simulink model "acdcmg_sim8_1_sm_grid_simulation"  (R2019b)
settings: Solver=ode8  StartTime=0.0  StopTime=0.5  FixedStep=4e-05  MaxStep=1e-2  RelTol=1e-3
PreLoadFcn:
  | Set_parameters_R2018
InitFcn:
  | Set_parameters_R2018
undefined symbols (not defined in the file or in its folder): D1, Delta, dis11, dis12, dis2, dis3, dis4, dis5, dis6, DiscIntNeverNeededParam, fn, Fnom, Ion, Lithium, max_min, P_Load_3, Pnom_T1, Pnom_T2, Pnom_T3, Ql_Load_3, R_Load_9, R_Load_DC, Rl, Rls, Ts, Ts_Control, Ts_Power, Ts_PV, V1_LL_T3, Vmin_mppt, VnInv, Vnom_DC, Vnom_Diesel, Vnom_prim, Vnom_sec, Vnom_ter_AC_DC, Xl, Xls
libraries: powerlib x136, powerlib_meascontrol x67, opal_lib x24, artemis x7, simulink x7, powerlib_extras x5, electricdrivelib x1, eeSinusoidalMeasurementV2 x1, re_lib x1
(part 2 of 4)

== system acdcmg_sim8_1_sm_grid_simulation/SM_Grid_Simulation/Bus_1 ==
  Mux : Mux  Inputs=2
  "Power (3ph, Instantaneous)" : powerlib_meascontrol/Measurements/Power (3ph, Instantaneous)
  Power Factor Block1 : Subsystem  mask(Power Factor Block){Freq=Fnom, Vinit=[0, 0], Iinit=[0, 0], Ts=0}
      mask prompts: Freq "Fundamental frequency (Hz):"; Vinit "Voltage initial input [ Mag, Phase (degrees) ]:"; Iinit "Current initial input [ Mag, Phase (degrees) ]:"; Ts "Sample time:"
      mask help:
      | Power Factor Block developed by Dr Rodney Tan
      | Version 1.01 (Aug 2016)
      |
      | Compute power factor and phase angle of AC circuit voltage-current pair at fundamental frequency.
      |
      | The computation is based on Power block and Complex number function block.
      |
      | For the first cycle of simulation, the outputs are held constant to the powers computed for the Voltage initial input and Current initial input parameters.
      mask Help:
      | <b>Fundamental Frequency (Hz)</b>
      | Specify the measurement fundamental frequency, in hertz, of the input signal.
      | 
      | <b>Voltage initial input [ Mag, Phase (degrees) ]</b>
      | Specify the voltage initial magnitude and phase to set a constant output for the first cycle of simulation.
      | 
      | <b>Current initial input [ Mag, Phase (degrees) ]</b>
      | Specify the current initial magnitude and phase to set a constant output for the first cycle of simulation.
      | 
      | <b>Sample Time</b>
      | Specify the sample time of the block, in seconds. Set to 0 to implement a continuous block.
      mask TypeOptions Freq: Power/Freq
      mask TypeOptions Vinit: Power/Vinit
      mask TypeOptions Iinit: Power/Iinit
      mask TypeOptions Ts: Power/Ts
  "Means_Bus1      " : Outport  VectorParamsAs1DForOutWhenUnconnected=off
  tag scope: Bus1_Iabc=global, Bus1_P=global, Bus1_Q=global, Bus1_Vabc=global
  wires:
  [IabcLL_Bus_1] -> "Power (3ph, Instantaneous)"/2, Power Factor Block1/2(Iabc), Mux/2  "Iabc"
  Mux/1 -> "Means_Bus1      "/1
  Power Factor Block1/2("Iabc y Iabc ") -> [Bus1_Iabc]
  Power Factor Block1/1("Vabc y Vabc ") -> [Bus1_Vabc]
  [VabcLL_Bus_1] -> Power Factor Block1/1(Vabc), "Power (3ph, Instantaneous)"/1, Mux/1  "Vabc"
  "Power (3ph, Instantaneous)"/1 -> [Bus1_P]
  "Power (3ph, Instantaneous)"/2 -> [Bus1_Q]

== system acdcmg_sim8_1_sm_grid_simulation/SM_Grid_Simulation/Bus_14 1 ==
  " r1_ L13" : Constant  Value=Rl
  Active powers losses A : Display
      settings: Format=bank
  Active powers losses B : Display
      settings: Format=bank
  Active powers losses c : Display
      settings: Format=bank
  Math Function : Math  Operator=square  SaturateOnIntegerOverflow=on
  Math Function1 : Math  Operator=square  SaturateOnIntegerOverflow=on
  Math Function2 : Math  Operator=square  SaturateOnIntegerOverflow=on
  Mux : Mux  Inputs=3
  Product : Product
  Product1 : Product
  Product2 : Product
  RMS1 : powerlib_meascontrol/Measurements/RMS  TrueRMS=on  Freq=60  RMSInit=0  Ts=0
  RMS2 : powerlib_meascontrol/Measurements/RMS  TrueRMS=on  Freq=60  RMSInit=0  Ts=0
  RMS3 : powerlib_meascontrol/Measurements/RMS  TrueRMS=on  Freq=60  RMSInit=0  Ts=0
  W_to_kW : Gain  Gain=1e-3
  W_to_kW1 : Gain  Gain=1e-3
  W_to_kW2 : Gain  Gain=1e-3
  tag scope: Bus_14_1_LineA_Ploss=global, Bus_14_1_LineB_Ploss=global, Bus_14_1_LineC_Ploss=global, Power_Losse_abc_L1=global
  wires:
  Math Function/1 -> Product/2
  [Ia_L1] -> RMS2/1
  Math Function1/1 -> Product1/2
  [Ib_L1] -> RMS1/1
  Math Function2/1 -> Product2/2
  " r1_ L13"/1 -> Product2/1, Product1/1, Product/1
  [Ic_L1] -> RMS3/1
  Product/1 -> W_to_kW/1
  Product2/1 -> W_to_kW2/1
  Product1/1 -> W_to_kW1/1
  RMS2/1 -> Math Function/1
  RMS1/1 -> Math Function1/1
  RMS3/1 -> Math Function2/1
  W_to_kW/1 -> [Bus_14_1_LineA_Ploss], Mux/1, Active powers losses A/1  "D_Pa_kW"
  W_to_kW1/1 -> [Bus_14_1_LineB_Ploss], Mux/2, Active powers losses B/1  "D_Pb_kW"
  W_to_kW2/1 -> Active powers losses c/1, [Bus_14_1_LineC_Ploss], Mux/3  "D_Pc_kW"
  Mux/1 -> [Power_Losse_abc_L1]

== system acdcmg_sim8_1_sm_grid_simulation/SM_Grid_Simulation/Bus_14 2 ==
  " r1_ L13" : Constant  Value=Rls
  Active powers losses A : Display
      settings: Format=bank
  Active powers losses B : Display
      settings: Format=bank
  Active powers losses c : Display
      settings: Format=bank
  Math Function : Math  Operator=square  SaturateOnIntegerOverflow=on
  Math Function1 : Math  Operator=square  SaturateOnIntegerOverflow=on
  Math Function2 : Math  Operator=square  SaturateOnIntegerOverflow=on
  Mux : Mux  Inputs=3
  Product : Product
  Product1 : Product
  Product2 : Product
  RMS1 : powerlib_meascontrol/Measurements/RMS  TrueRMS=on  Freq=60  RMSInit=0  Ts=0
  RMS2 : powerlib_meascontrol/Measurements/RMS  TrueRMS=on  Freq=60  RMSInit=0  Ts=0
  RMS3 : powerlib_meascontrol/Measurements/RMS  TrueRMS=on  Freq=60  RMSInit=0  Ts=0
  W_to_kW : Gain  Gain=1e-3
  W_to_kW1 : Gain  Gain=1e-3
  W_to_kW2 : Gain  Gain=1e-3
  tag scope: Bus_14_2_LineA_Ploss=global, Bus_14_2_LineB_Ploss=global, Bus_14_2_LineC_Ploss=global, Power_Losse_abc_L2=global
  wires:
  Math Function/1 -> Product/2
  [Ia_L2] -> RMS2/1
  Math Function1/1 -> Product1/2
  [Ib_L2] -> RMS1/1
  Math Function2/1 -> Product2/2
  " r1_ L13"/1 -> Product2/1, Product1/1, Product/1
  [Ic_L2] -> RMS3/1
  Product/1 -> W_to_kW/1
  Product2/1 -> W_to_kW2/1
  Product1/1 -> W_to_kW1/1
  RMS2/1 -> Math Function/1
  RMS1/1 -> Math Function1/1
  RMS3/1 -> Math Function2/1
  W_to_kW/1 -> [Bus_14_2_LineA_Ploss], Mux/1, Active powers losses A/1  "D_Pa_kW"
  W_to_kW1/1 -> [Bus_14_2_LineB_Ploss], Mux/2, Active powers losses B/1  "D_Pb_kW"
  W_to_kW2/1 -> Active powers losses c/1, [Bus_14_2_LineC_Ploss], Mux/3  "D_Pc_kW"
  Mux/1 -> [Power_Losse_abc_L2]

== system acdcmg_sim8_1_sm_grid_simulation/SM_Grid_Simulation/Bus_14 3 ==
  " r1_ L13" : Constant  Value=Rl
  Active powers losses A : Display  Commented=on
      settings: Format=bank
  Active powers losses B : Display  Commented=on
      settings: Format=bank
  Active powers losses c : Display  Commented=on
      settings: Format=bank
  "Delta Pabc " : Scope  NumInputPorts=4
  Math Function : Math  Operator=square  SaturateOnIntegerOverflow=on
  Math Function1 : Math  Operator=square  SaturateOnIntegerOverflow=on
  Math Function2 : Math  Operator=square  SaturateOnIntegerOverflow=on
  Mux : Mux  Inputs=3
  Product : Product
  Product1 : Product
  Product2 : Product
  RMS1 : powerlib_meascontrol/Measurements/RMS  TrueRMS=on  Freq=60  RMSInit=0  Ts=0
  RMS2 : powerlib_meascontrol/Measurements/RMS  TrueRMS=on  Freq=60  RMSInit=0  Ts=0
  RMS3 : powerlib_meascontrol/Measurements/RMS  TrueRMS=on  Freq=60  RMSInit=0  Ts=0
  W_to_kW : Gain  Gain=1e-3
  W_to_kW1 : Gain  Gain=1e-3
  W_to_kW2 : Gain  Gain=1e-3
  tag scope: Bus_14_3_LineA_Ploss=global, Bus_14_3_LineB_Ploss=global, Bus_14_3_LineC_Ploss=global, Power_Losse_abc_L3=global
  wires:
  Math Function/1 -> Product/2
  [Ia_L3] -> RMS2/1
  Math Function1/1 -> Product1/2
  [Ib_L3] -> RMS1/1
  Math Function2/1 -> Product2/2
  " r1_ L13"/1 -> Product2/1, Product1/1, Product/1
  [Ic_L3] -> RMS3/1
  Product/1 -> W_to_kW/1
  Product2/1 -> W_to_kW2/1
  Product1/1 -> W_to_kW1/1
  RMS2/1 -> Math Function/1
  RMS1/1 -> Math Function1/1
  RMS3/1 -> Math Function2/1
  W_to_kW/1 -> Mux/1, [Bus_14_3_LineA_Ploss], Active powers losses A/1  "D_Pa_kW"
  W_to_kW1/1 -> Mux/2, [Bus_14_3_LineB_Ploss], Active powers losses B/1  "D_Pb_kW"
  W_to_kW2/1 -> Active powers losses c/1, Mux/3, [Bus_14_3_LineC_Ploss]  "D_Pc_kW"
  Mux/1 -> [Power_Losse_abc_L3]

== system acdcmg_sim8_1_sm_grid_simulation/SM_Grid_Simulation/Bus_14 4 ==
  " r1_ L13" : Constant  Value=Rls
  Active powers losses A : Display
      settings: Format=bank
  Active powers losses B : Display
      settings: Format=bank
  Active powers losses c : Display
      settings: Format=bank
  Math Function : Math  Operator=square  SaturateOnIntegerOverflow=on
  Math Function1 : Math  Operator=square  SaturateOnIntegerOverflow=on
  Math Function2 : Math  Operator=square  SaturateOnIntegerOverflow=on
  Mux : Mux  Inputs=3
  Product : Product
  Product1 : Product
  Product2 : Product
  RMS1 : powerlib_meascontrol/Measurements/RMS  TrueRMS=on  Freq=60  RMSInit=0  Ts=0
  RMS2 : powerlib_meascontrol/Measurements/RMS  TrueRMS=on  Freq=60  RMSInit=0  Ts=0
  RMS3 : powerlib_meascontrol/Measurements/RMS  TrueRMS=on  Freq=60  RMSInit=0  Ts=0
  W_to_kW : Gain  Gain=1e-3
  W_to_kW1 : Gain  Gain=1e-3
  W_to_kW2 : Gain  Gain=1e-3
  tag scope: Bus_14_4_LineA_Ploss=global, Bus_14_4_LineB_Ploss=global, Bus_14_4_LineC_Ploss=global, Power_Losse_abc_L4=global
  wires:
  Math Function/1 -> Product/2
  [Ia_L4] -> RMS2/1
  Math Function1/1 -> Product1/2
  [Ib_L4] -> RMS1/1
  Math Function2/1 -> Product2/2
  " r1_ L13"/1 -> Product2/1, Product1/1, Product/1
  [Ic_L4] -> RMS3/1
  Product/1 -> W_to_kW/1
  Product2/1 -> W_to_kW2/1
  Product1/1 -> W_to_kW1/1
  RMS2/1 -> Math Function/1
  RMS1/1 -> Math Function1/1
  RMS3/1 -> Math Function2/1
  W_to_kW/1 -> Mux/1, [Bus_14_4_LineA_Ploss], Active powers losses A/1  "D_Pa_kW"
  W_to_kW1/1 -> Mux/2, [Bus_14_4_LineB_Ploss], Active powers losses B/1  "D_Pb_kW"
  W_to_kW2/1 -> Active powers losses c/1, [Bus_14_4_LineC_Ploss], Mux/3  "D_Pc_kW"
  Mux/1 -> [Power_Losse_abc_L4]

== system acdcmg_sim8_1_sm_grid_simulation/SM_Grid_Simulation/Bus_14 5 ==
  " r1_ L13" : Constant  Value=Rls
  Active powers losses A : Display
      settings: Format=bank
  Active powers losses B : Display
      settings: Format=bank
  Active powers losses c : Display
      settings: Format=bank
  Math Function : Math  Operator=square  SaturateOnIntegerOverflow=on
  Math Function1 : Math  Operator=square  SaturateOnIntegerOverflow=on
  Math Function2 : Math  Operator=square  SaturateOnIntegerOverflow=on
  Mux : Mux  Inputs=3
  Product : Product
  Product1 : Product
  Product2 : Product
  RMS1 : powerlib_meascontrol/Measurements/RMS  TrueRMS=on  Freq=60  RMSInit=0  Ts=0
  RMS2 : powerlib_meascontrol/Measurements/RMS  TrueRMS=on  Freq=60  RMSInit=0  Ts=0
  RMS3 : powerlib_meascontrol/Measurements/RMS  TrueRMS=on  Freq=60  RMSInit=0  Ts=0
  W_to_kW : Gain  Gain=1e-3
  W_to_kW1 : Gain  Gain=1e-3
  W_to_kW2 : Gain  Gain=1e-3
  tag scope: Bus_14_5_LineA_Ploss=global, Bus_14_5_LineB_Ploss=global, Bus_14_5_LineC_Ploss=global, Power_Losse_abc_L5=global
  wires:
  Math Function/1 -> Product/2
  [Ia_L5] -> RMS2/1
  Math Function1/1 -> Product1/2
  [Ib_L5] -> RMS1/1
  Math Function2/1 -> Product2/2
  " r1_ L13"/1 -> Product2/1, Product1/1, Product/1
  [Ic_L5] -> RMS3/1
  Product/1 -> W_to_kW/1
  Product2/1 -> W_to_kW2/1
  Product1/1 -> W_to_kW1/1
  RMS2/1 -> Math Function/1
  RMS1/1 -> Math Function1/1
  RMS3/1 -> Math Function2/1
  W_to_kW/1 -> [Bus_14_5_LineA_Ploss], Mux/1, Active powers losses A/1  "D_Pa_kW"
  W_to_kW1/1 -> [Bus_14_5_LineB_Ploss], Mux/2, Active powers losses B/1  "D_Pb_kW"
  W_to_kW2/1 -> Active powers losses c/1, [Bus_14_5_LineC_Ploss], Mux/3  "D_Pc_kW"
  Mux/1 -> [Power_Losse_abc_L5]

== system acdcmg_sim8_1_sm_grid_simulation/SM_Grid_Simulation/Bus_14 6 ==
  " r1_ L13" : Constant  Value=Rls
  Active powers losses A : Display
      settings: Format=bank
  Active powers losses B : Display
      settings: Format=bank
  Active powers losses c : Display
      settings: Format=bank
  Math Function : Math  Operator=square  SaturateOnIntegerOverflow=on
  Math Function1 : Math  Operator=square  SaturateOnIntegerOverflow=on
  Math Function2 : Math  Operator=square  SaturateOnIntegerOverflow=on
  Mux : Mux  Inputs=3
  Product : Product
  Product1 : Product
  Product2 : Product
  RMS1 : powerlib_meascontrol/Measurements/RMS  TrueRMS=on  Freq=60  RMSInit=0  Ts=0
  RMS2 : powerlib_meascontrol/Measurements/RMS  TrueRMS=on  Freq=60  RMSInit=0  Ts=0
  RMS3 : powerlib_meascontrol/Measurements/RMS  TrueRMS=on  Freq=60  RMSInit=0  Ts=0
  W_to_kW : Gain  Gain=1e-3
  W_to_kW1 : Gain  Gain=1e-3
  W_to_kW2 : Gain  Gain=1e-3
  tag scope: Bus_14_6_LineA_Ploss=global, Bus_14_6_LineB_Ploss=global, Bus_14_6_LineC_Ploss=global, Power_Losse_abc_L6=global
  wires:
  Math Function/1 -> Product/2
  [Ia_L6] -> RMS2/1
  Math Function1/1 -> Product1/2
  [Ib_L6] -> RMS1/1
  Math Function2/1 -> Product2/2
  " r1_ L13"/1 -> Product2/1, Product1/1, Product/1
  [Ic_L6] -> RMS3/1
  Product/1 -> W_to_kW/1
  Product2/1 -> W_to_kW2/1
  Product1/1 -> W_to_kW1/1
  RMS2/1 -> Math Function/1
  RMS1/1 -> Math Function1/1
  RMS3/1 -> Math Function2/1
  W_to_kW/1 -> [Bus_14_6_LineA_Ploss], Mux/1, Active powers losses A/1  "D_Pa_kW"
  W_to_kW1/1 -> [Bus_14_6_LineB_Ploss], Mux/2, Active powers losses B/1  "D_Pb_kW"
  W_to_kW2/1 -> Active powers losses c/1, [Bus_14_6_LineC_Ploss], Mux/3  "D_Pc_kW"
  Mux/1 -> [Power_Losse_abc_L6]

== system acdcmg_sim8_1_sm_grid_simulation/SM_Grid_Simulation/Bus_14 7 ==
  " r1_ L13" : Constant  Value=Rls
  Active powers losses A : Display
      settings: Format=bank
  Active powers losses B : Display
      settings: Format=bank
  Active powers losses c : Display
      settings: Format=bank
  Math Function : Math  Operator=square  SaturateOnIntegerOverflow=on
  Math Function1 : Math  Operator=square  SaturateOnIntegerOverflow=on
  Math Function2 : Math  Operator=square  SaturateOnIntegerOverflow=on
  Mux : Mux  Inputs=3
  Product : Product
  Product1 : Product
  Product2 : Product
  RMS1 : powerlib_meascontrol/Measurements/RMS  TrueRMS=on  Freq=60  RMSInit=0  Ts=0
  RMS2 : powerlib_meascontrol/Measurements/RMS  TrueRMS=on  Freq=60  RMSInit=0  Ts=0
  RMS3 : powerlib_meascontrol/Measurements/RMS  TrueRMS=on  Freq=60  RMSInit=0  Ts=0
  W_to_kW : Gain  Gain=1e-3
  W_to_kW1 : Gain  Gain=1e-3
  W_to_kW2 : Gain  Gain=1e-3
  tag scope: Bus_14_7_LineA_Ploss=global, Bus_14_7_LineB_Ploss=global, Bus_14_7_LineC_Ploss=global, Power_Losse_abc_L7=global
  wires:
  Math Function/1 -> Product/2
  [Ia_L7] -> RMS2/1
  Math Function1/1 -> Product1/2
  [Ib_L7] -> RMS1/1
  Math Function2/1 -> Product2/2
  " r1_ L13"/1 -> Product2/1, Product1/1, Product/1
  [Ic_L7] -> RMS3/1
  Product/1 -> W_to_kW/1
  Product2/1 -> W_to_kW2/1
  Product1/1 -> W_to_kW1/1
  RMS2/1 -> Math Function/1
  RMS1/1 -> Math Function1/1
  RMS3/1 -> Math Function2/1
  W_to_kW/1 -> [Bus_14_7_LineA_Ploss], Mux/1, Active powers losses A/1  "D_Pa_kW"
  W_to_kW1/1 -> [Bus_14_7_LineB_Ploss], Mux/2, Active powers losses B/1  "D_Pb_kW"
  W_to_kW2/1 -> Active powers losses c/1, [Bus_14_7_LineC_Ploss], Mux/3  "D_Pc_kW"
  Mux/1 -> [Power_Losse_abc_L7]

== system acdcmg_sim8_1_sm_grid_simulation/SM_Grid_Simulation/Bus_2 ==
  "Power (3ph, Instantaneous)" : powerlib_meascontrol/Measurements/Power (3ph, Instantaneous)
  Power Factor Block1 : Subsystem  mask(Power Factor Block){Freq=Fnom, Vinit=[0, 0], Iinit=[0, 0], Ts=0}
      mask prompts: Freq "Fundamental frequency (Hz):"; Vinit "Voltage initial input [ Mag, Phase (degrees) ]:"; Iinit "Current initial input [ Mag, Phase (degrees) ]:"; Ts "Sample time:"
      mask help:
      | Power Factor Block developed by Dr Rodney Tan
      | Version 1.01 (Aug 2016)
      |
      | Compute power factor and phase angle of AC circuit voltage-current pair at fundamental frequency.
      |
      | The computation is based on Power block and Complex number function block.
      |
      | For the first cycle of simulation, the outputs are held constant to the powers computed for the Voltage initial input and Current initial input parameters.
      mask Help:
      | <b>Fundamental Frequency (Hz)</b>
      | Specify the measurement fundamental frequency, in hertz, of the input signal.
      | 
      | <b>Voltage initial input [ Mag, Phase (degrees) ]</b>
      | Specify the voltage initial magnitude and phase to set a constant output for the first cycle of simulation.
      | 
      | <b>Current initial input [ Mag, Phase (degrees) ]</b>
      | Specify the current initial magnitude and phase to set a constant output for the first cycle of simulation.
      | 
      | <b>Sample Time</b>
      | Specify the sample time of the block, in seconds. Set to 0 to implement a continuous block.
      mask TypeOptions Freq: Power/Freq
      mask TypeOptions Vinit: Power/Vinit
      mask TypeOptions Iinit: Power/Iinit
      mask TypeOptions Ts: Power/Ts
  tag scope: Bus2_Iabc=global, Bus2_P=global, Bus2_Q=global, Bus2_Vabc=global
  wires:
  [IabcLL_Bus_2] -> "Power (3ph, Instantaneous)"/2, Power Factor Block1/2(Iabc)
  [VabcLL_Bus_2] -> "Power (3ph, Instantaneous)"/1, Power Factor Block1/1(Vabc)  "Vabc"
  "Power (3ph, Instantaneous)"/1 -> [Bus2_P]
  "Power (3ph, Instantaneous)"/2 -> [Bus2_Q]
  Power Factor Block1/1("Vabc y Vabc ") -> [Bus2_Vabc]
  Power Factor Block1/2("Iabc y Iabc ") -> [Bus2_Iabc]

== system acdcmg_sim8_1_sm_grid_simulation/SM_Grid_Simulation/Bus_3 ==
  "Power (3ph, Instantaneous)" : powerlib_meascontrol/Measurements/Power (3ph, Instantaneous)
  Power Factor Block1 : Subsystem  mask(Power Factor Block){Freq=Fnom, Vinit=[0, 0], Iinit=[0, 0], Ts=0}
      mask prompts: Freq "Fundamental frequency (Hz):"; Vinit "Voltage initial input [ Mag, Phase (degrees) ]:"; Iinit "Current initial input [ Mag, Phase (degrees) ]:"; Ts "Sample time:"
      mask help:
      | Power Factor Block developed by Dr Rodney Tan
      | Version 1.01 (Aug 2016)
      |
      | Compute power factor and phase angle of AC circuit voltage-current pair at fundamental frequency.
      |
      | The computation is based on Power block and Complex number function block.
      |
      | For the first cycle of simulation, the outputs are held constant to the powers computed for the Voltage initial input and Current initial input parameters.
      mask Help:
      | <b>Fundamental Frequency (Hz)</b>
      | Specify the measurement fundamental frequency, in hertz, of the input signal.
      | 
      | <b>Voltage initial input [ Mag, Phase (degrees) ]</b>
      | Specify the voltage initial magnitude and phase to set a constant output for the first cycle of simulation.
      | 
      | <b>Current initial input [ Mag, Phase (degrees) ]</b>
      | Specify the current initial magnitude and phase to set a constant output for the first cycle of simulation.
      | 
      | <b>Sample Time</b>
      | Specify the sample time of the block, in seconds. Set to 0 to implement a continuous block.
      mask TypeOptions Freq: Power/Freq
      mask TypeOptions Vinit: Power/Vinit
      mask TypeOptions Iinit: Power/Iinit
      mask TypeOptions Ts: Power/Ts
  tag scope: Bus3_Iabc=global, Bus3_P=global, Bus3_Q=global, Bus3_Vabc=global
  wires:
  [IabcLL_Bus_3] -> "Power (3ph, Instantaneous)"/2, Power Factor Block1/2(Iabc)
  [VabcLL_Bus_3] -> "Power (3ph, Instantaneous)"/1, Power Factor Block1/1(Vabc)  "Signal Vabc"
  "Power (3ph, Instantaneous)"/1 -> [Bus3_P]
  "Power (3ph, Instantaneous)"/2 -> [Bus3_Q]
  Power Factor Block1/1(Vabc y Vabc) -> [Bus3_Vabc]
  Power Factor Block1/2("Iabc y Iabc ") -> [Bus3_Iabc]

== system acdcmg_sim8_1_sm_grid_simulation/SM_Grid_Simulation/Bus_4 ==
  "Power (3ph, Instantaneous)" : powerlib_meascontrol/Measurements/Power (3ph, Instantaneous)
  Power Factor Block1 : Subsystem  mask(Power Factor Block){Freq=Fnom, Vinit=[0, 0], Iinit=[0, 0], Ts=0}
      mask prompts: Freq "Fundamental frequency (Hz):"; Vinit "Voltage initial input [ Mag, Phase (degrees) ]:"; Iinit "Current initial input [ Mag, Phase (degrees) ]:"; Ts "Sample time:"
      mask help:
      | Power Factor Block developed by Dr Rodney Tan
      | Version 1.01 (Aug 2016)
      |
      | Compute power factor and phase angle of AC circuit voltage-current pair at fundamental frequency.
      |
      | The computation is based on Power block and Complex number function block.
      |
      | For the first cycle of simulation, the outputs are held constant to the powers computed for the Voltage initial input and Current initial input parameters.
      mask Help:
      | <b>Fundamental Frequency (Hz)</b>
      | Specify the measurement fundamental frequency, in hertz, of the input signal.
      | 
      | <b>Voltage initial input [ Mag, Phase (degrees) ]</b>
      | Specify the voltage initial magnitude and phase to set a constant output for the first cycle of simulation.
      | 
      | <b>Current initial input [ Mag, Phase (degrees) ]</b>
      | Specify the current initial magnitude and phase to set a constant output for the first cycle of simulation.
      | 
      | <b>Sample Time</b>
      | Specify the sample time of the block, in seconds. Set to 0 to implement a continuous block.
      mask TypeOptions Freq: Power/Freq
      mask TypeOptions Vinit: Power/Vinit
      mask TypeOptions Iinit: Power/Iinit
      mask TypeOptions Ts: Power/Ts
  tag scope: Bus4_Iabc=global, Bus4_P=global, Bus4_Q=global, Bus4_Vabc=global
  wires:
  [IabcLL_Bus_4] -> "Power (3ph, Instantaneous)"/2, Power Factor Block1/2(Iabc)
  Power Factor Block1/2("Iabc y Iabc ") -> [Bus4_Iabc]
  Power Factor Block1/1(Vabc y Vabc) -> [Bus4_Vabc]
  [VabcLL_Bus_4] -> "Power (3ph, Instantaneous)"/1, Power Factor Block1/1(Vabc)  "Signal Vabc"
  "Power (3ph, Instantaneous)"/1 -> [Bus4_P]
  "Power (3ph, Instantaneous)"/2 -> [Bus4_Q]

== system acdcmg_sim8_1_sm_grid_simulation/SM_Grid_Simulation/Bus_5 ==
  "Power (3ph, Instantaneous)" : powerlib_meascontrol/Measurements/Power (3ph, Instantaneous)
  Power Factor Block1 : Subsystem  mask(Power Factor Block){Freq=Fnom, Vinit=[0, 0], Iinit=[0, 0], Ts=0}
      mask prompts: Freq "Fundamental frequency (Hz):"; Vinit "Voltage initial input [ Mag, Phase (degrees) ]:"; Iinit "Current initial input [ Mag, Phase (degrees) ]:"; Ts "Sample time:"
      mask help:
      | Power Factor Block developed by Dr Rodney Tan
      | Version 1.01 (Aug 2016)
      |
      | Compute power factor and phase angle of AC circuit voltage-current pair at fundamental frequency.
      |
      | The computation is based on Power block and Complex number function block.
      |
      | For the first cycle of simulation, the outputs are held constant to the powers computed for the Voltage initial input and Current initial input parameters.
      mask Help:
      | <b>Fundamental Frequency (Hz)</b>
      | Specify the measurement fundamental frequency, in hertz, of the input signal.
      | 
      | <b>Voltage initial input [ Mag, Phase (degrees) ]</b>
      | Specify the voltage initial magnitude and phase to set a constant output for the first cycle of simulation.
      | 
      | <b>Current initial input [ Mag, Phase (degrees) ]</b>
      | Specify the current initial magnitude and phase to set a constant output for the first cycle of simulation.
      | 
      | <b>Sample Time</b>
      | Specify the sample time of the block, in seconds. Set to 0 to implement a continuous block.
      mask TypeOptions Freq: Power/Freq
      mask TypeOptions Vinit: Power/Vinit
      mask TypeOptions Iinit: Power/Iinit
      mask TypeOptions Ts: Power/Ts
  tag scope: Bus5_Iabc=global, Bus5_P=global, Bus5_Q=global, Bus5_Vabc=global
  wires:
  [IabcLL_Bus_5] -> Power Factor Block1/2(Iabc), "Power (3ph, Instantaneous)"/2
  Power Factor Block1/2("Iabc y Iabc ") -> [Bus5_Iabc]
  Power Factor Block1/1(Vabc y Vabc) -> [Bus5_Vabc]
  [VabcLL_Bus_5] -> "Power (3ph, Instantaneous)"/1, Power Factor Block1/1(Vabc)  "Signal Vabc"
  "Power (3ph, Instantaneous)"/1 -> [Bus5_P]
  "Power (3ph, Instantaneous)"/2 -> [Bus5_Q]

== system acdcmg_sim8_1_sm_grid_simulation/SM_Grid_Simulation/Bus_6 ==
  "Power (3ph, Instantaneous)" : powerlib_meascontrol/Measurements/Power (3ph, Instantaneous)
  Power Factor Block1 : Subsystem  mask(Power Factor Block){Freq=Fnom, Vinit=[0, 0], Iinit=[0, 0], Ts=0}
      mask prompts: Freq "Fundamental frequency (Hz):"; Vinit "Voltage initial input [ Mag, Phase (degrees) ]:"; Iinit "Current initial input [ Mag, Phase (degrees) ]:"; Ts "Sample time:"
      mask help:
      | Power Factor Block developed by Dr Rodney Tan
      | Version 1.01 (Aug 2016)
      |
      | Compute power factor and phase angle of AC circuit voltage-current pair at fundamental frequency.
      |
      | The computation is based on Power block and Complex number function block.
      |
      | For the first cycle of simulation, the outputs are held constant to the powers computed for the Voltage initial input and Current initial input parameters.
      mask Help:
      | <b>Fundamental Frequency (Hz)</b>
      | Specify the measurement fundamental frequency, in hertz, of the input signal.
      | 
      | <b>Voltage initial input [ Mag, Phase (degrees) ]</b>
      | Specify the voltage initial magnitude and phase to set a constant output for the first cycle of simulation.
      | 
      | <b>Current initial input [ Mag, Phase (degrees) ]</b>
      | Specify the current initial magnitude and phase to set a constant output for the first cycle of simulation.
      | 
      | <b>Sample Time</b>
      | Specify the sample time of the block, in seconds. Set to 0 to implement a continuous block.
      mask TypeOptions Freq: Power/Freq
      mask TypeOptions Vinit: Power/Vinit
      mask TypeOptions Iinit: Power/Iinit
      mask TypeOptions Ts: Power/Ts
  tag scope: Bus6_Iabc=global, Bus6_P=global, Bus6_Q=global, Bus6_Vabc=global
  wires:
  [IabcLL_Bus_6] -> Power Factor Block1/2(Iabc), "Power (3ph, Instantaneous)"/2
  Power Factor Block1/1("Vabc y Vabc ") -> [Bus6_Vabc]
  Power Factor Block1/2(Iabc y Iabc) -> [Bus6_Iabc]
  [VabcLL_Bus_6] -> "Power (3ph, Instantaneous)"/1, Power Factor Block1/1(Vabc)  "Vabc"
  "Power (3ph, Instantaneous)"/1 -> [Bus6_P]
  "Power (3ph, Instantaneous)"/2 -> [Bus6_Q]

== system acdcmg_sim8_1_sm_grid_simulation/SM_Grid_Simulation/Bus_7 ==
  "Power (3ph, Instantaneous)" : powerlib_meascontrol/Measurements/Power (3ph, Instantaneous)
  Power Factor Block1 : Subsystem  mask(Power Factor Block){Freq=Fnom, Vinit=[0, 0], Iinit=[0, 0], Ts=0}
      mask prompts: Freq "Fundamental frequency (Hz):"; Vinit "Voltage initial input [ Mag, Phase (degrees) ]:"; Iinit "Current initial input [ Mag, Phase (degrees) ]:"; Ts "Sample time:"
      mask help:
      | Power Factor Block developed by Dr Rodney Tan
      | Version 1.01 (Aug 2016)
      |
      | Compute power factor and phase angle of AC circuit voltage-current pair at fundamental frequency.
      |
      | The computation is based on Power block and Complex number function block.
      |
      | For the first cycle of simulation, the outputs are held constant to the powers computed for the Voltage initial input and Current initial input parameters.
      mask Help:
      | <b>Fundamental Frequency (Hz)</b>
      | Specify the measurement fundamental frequency, in hertz, of the input signal.
      | 
      | <b>Voltage initial input [ Mag, Phase (degrees) ]</b>
      | Specify the voltage initial magnitude and phase to set a constant output for the first cycle of simulation.
      | 
      | <b>Current initial input [ Mag, Phase (degrees) ]</b>
      | Specify the current initial magnitude and phase to set a constant output for the first cycle of simulation.
      | 
      | <b>Sample Time</b>
      | Specify the sample time of the block, in seconds. Set to 0 to implement a continuous block.
      mask TypeOptions Freq: Power/Freq
      mask TypeOptions Vinit: Power/Vinit
      mask TypeOptions Iinit: Power/Iinit
      mask TypeOptions Ts: Power/Ts
  tag scope: Bus7_Iabc=global, Bus7_P=global, Bus7_Q=global, Bus7_Vabc=global
  wires:
  [IabcLL_Bus_7] -> "Power (3ph, Instantaneous)"/2, Power Factor Block1/2(Iabc)
  [VabcLL_Bus_7] -> "Power (3ph, Instantaneous)"/1, Power Factor Block1/1(Vabc)  "Signal Vabc"
  Power Factor Block1/1(Vabc y Vabc) -> [Bus7_Vabc]
  Power Factor Block1/2("Iabc y Iabc ") -> [Bus7_Iabc]
  "Power (3ph, Instantaneous)"/2 -> [Bus7_Q]
  "Power (3ph, Instantaneous)"/1 -> [Bus7_P]

== system acdcmg_sim8_1_sm_grid_simulation/SM_Grid_Simulation/Bus_8 ==
  Gain2 : Gain  Commented=on  Gain=Fnom
  Goto2 : Goto  Commented=on  GotoTag=w_iv  TagVisibility=global
  "PMU (PLL-Based, Positive-Sequence)" : powerlib_meascontrol/Measurements/PMU (PLL-Based, Positive-Sequence)  Commented=on  nominalFrequency=60  samplingRate=24  reportingFactor=1
      settings: SourceProductBaseCode=PS
  "Power (3ph, Instantaneous)" : powerlib_meascontrol/Measurements/Power (3ph, Instantaneous)
  Power Factor Block1 : Subsystem  mask(Power Factor Block){Freq=1/Ts, Vinit=[0, 0], Iinit=[0, 0], Ts=Ts}
      mask prompts: Freq "Fundamental frequency (Hz):"; Vinit "Voltage initial input [ Mag, Phase (degrees) ]:"; Iinit "Current initial input [ Mag, Phase (degrees) ]:"; Ts "Sample time:"
      mask help:
      | Power Factor Block developed by Dr Rodney Tan
      | Version 1.01 (Aug 2016)
      |
      | Compute power factor and phase angle of AC circuit voltage-current pair at fundamental frequency.
      |
      | The computation is based on Power block and Complex number function block.
      |
      | For the first cycle of simulation, the outputs are held constant to the powers computed for the Voltage initial input and Current initial input parameters.
      mask Help:
      | <b>Fundamental Frequency (Hz)</b>
      | Specify the measurement fundamental frequency, in hertz, of the input signal.
      | 
      | <b>Voltage initial input [ Mag, Phase (degrees) ]</b>
      | Specify the voltage initial magnitude and phase to set a constant output for the first cycle of simulation.
      | 
      | <b>Current initial input [ Mag, Phase (degrees) ]</b>
      | Specify the current initial magnitude and phase to set a constant output for the first cycle of simulation.
      | 
      | <b>Sample Time</b>
      | Specify the sample time of the block, in seconds. Set to 0 to implement a continuous block.
      mask TypeOptions Freq: Power/Freq
      mask TypeOptions Vinit: Power/Vinit
      mask TypeOptions Iinit: Power/Iinit
      mask TypeOptions Ts: Power/Ts
  Scope4 : Scope  Commented=on  NumInputPorts=3
  "Sinusoidal Measurement (PLL, Three-Phase)1" : eeSinusoidalMeasurementV2/Sinusoidal Measurement (PLL, Three-Phase)  Commented=on  Kp_LF=Kp_pll  Ki_LF=Ki_pll  F0=60  Theta0=0  Ts=Ts
      settings: SourceProductName=Simscape Electrical  SourceProductBaseCode=PS
  tag scope: Bus8_Iabc=global, Bus8_P=global, Bus8_Q=global, Bus8_Vabc=global
  wires:
  [IabcLL_Bus_8] -> "Power (3ph, Instantaneous)"/2, Power Factor Block1/2(Iabc)
  [VabcLL_Bus_8] -> "Power (3ph, Instantaneous)"/1, Power Factor Block1/1(Vabc)  "Vabc"
  "PMU (PLL-Based, Positive-Sequence)"/3 -> Scope4/3
  "PMU (PLL-Based, Positive-Sequence)"/1 -> Gain2/1, Scope4/1
  Gain2/1 -> Goto2/1
  "PMU (PLL-Based, Positive-Sequence)"/2 -> Scope4/2
  "Power (3ph, Instantaneous)"/1 -> [Bus8_P]
  "Power (3ph, Instantaneous)"/2 -> [Bus8_Q]
  Power Factor Block1/1("Vabc y Vabc ") -> [Bus8_Vabc]
  Power Factor Block1/2("Iabc y Iabc ") -> [Bus8_Iabc]

== system acdcmg_sim8_1_sm_grid_simulation/SM_Grid_Simulation/Bus_AC//DC3 ==
  note: BUS
  Add : Sum
  Battery system : Subsystem
      mask Display: disp('Open this block\nto display additional \nscopes & measurements')
  Conv pu1 : Gain  Gain=1 /Vnom_DC  SaturateOnIntegerOverflow=on  OutDataTypeStr=Inherit: Same as input  ParamDataTypeStr=Inherit: Same as input
  Display : Display
  Display1 : Display
  Display6 : Display
  Gain : Gain  Gain=1/1000
  Mean : powerlib_meascontrol/Measurements/Mean  Freq=1/(Ts*2)  Vinit=0  Ts=0
  Memory : Memory
  Memory1 : Memory
  Mux : Mux  Inputs=1
  PV system : Subsystem
      mask Display: disp('Open this block\nto display additional \nscopes & measurements')
  Product : Product
  tag scope: DC_Bus_Power_kw=global, IDC_Bus=global, P_BusDC=global, V_pu_BusDC=global
  wires:
  Conv pu1/1 -> [VDC_Bus_pu], [V_pu_BusDC]  "DC Voltage (pu)"
  [V_DC_bus] -> Product/1, Conv pu1/1
  Mean/1 -> Mux/1, Product/2, Display6/1
  Product/1 -> Gain/1
  Mux/1 -> [IDC_Bus]
  Gain/1 -> [DC_Bus_Power_kw], [P_BusDC]  "Power (kW)"
  Add/1 -> Mean/1
  [I_DC_bus_PV] -> Memory1/1
  Memory1/1 -> Display1/1, Add/2
  [I_DC_bus_BESS] -> Memory/1
  Memory/1 -> Display/1, Add/1

== system acdcmg_sim8_1_sm_grid_simulation/SM_Grid_Simulation/DATA  ADQUISITION ==
  note: Transformer (T1)
  Power_Losses_abc : Subsystem
  VoltageLL_pu_abc : Subsystem
  scope 11 : Scope
  scope 12 : Scope
  wires:
  [Vabc_Sec_pu] -> scope 11/1
  [Vabc_Prim_pu] -> scope 12/1

== system acdcmg_sim8_1_sm_grid_simulation/SM_Grid_Simulation/Diesel_ 50MVA ==
  note: Diesel generator 2
  2.4kV  50MVA : powerlib/Elements/Three-Phase Series RLC Branch  LConnTagsString=A|B|C  RConnTagsString=A|B|C  BranchType=RL  Resistance=2.4e3^2/50e6/10  Inductance=2.4e3^2/50e6/(2*pi*60)  Capacitance=1.0  Measurements=None
  Ground1 : powerlib/Elements/Ground  LConnTagsString=a
  Programmable Voltage Source1 : powerlib/Electrical Sources/Three-Phase Programmable Voltage Source  PositiveSequence="[Vnom_Diesel*0.9848 -60  Fnom]"  VariationEntity=None  VariationType=Table of time-amplitude pairs  VariationTypeAlt=Step  VariationStep=-0.3  VariationRate=0.5  VariationMagnitude=0.4  VariationFrequency=2  VariationTiming=[0.1 1.2]  VariationPhaseA=off  Amplitudes=[1]  TimeValues=[0]  HarmonicGeneration=off  HarmonicA=[3 0.2 -25 0]  HarmonicB="[2 0.15  35 2]"  Timing="[0.1  0.6]"  BusType=PV  Pref=Pgen_Diesel  Qref=0  Qmin=-inf  Qmax=inf
  a1 : PMIOPort  Tag=PMCPort  Side=Left
  b1 : PMIOPort  Tag=PMCPort  Port=2  Side=Left
  c1 : PMIOPort  Tag=PMCPort  Port=3  Side=Left
  connections:
  Programmable Voltage Source1/RConn3 -- 2.4kV  50MVA/LConn3
  Ground1/LConn1 -- Programmable Voltage Source1/LConn1
  Programmable Voltage Source1/RConn2 -- 2.4kV  50MVA/LConn2
  2.4kV  50MVA/LConn1 -- Programmable Voltage Source1/RConn1
  b1/RConn1 -- 2.4kV  50MVA/RConn2
  a1/RConn1 -- 2.4kV  50MVA/RConn1
  c1/RConn1 -- 2.4kV  50MVA/RConn3

== system acdcmg_sim8_1_sm_grid_simulation/SM_Grid_Simulation/Grid Bi-directional Converter 1.1 300 (DC) // 150 V (AC) P_nom 3kW2 ==
  note: Bus DC
  note: Bus AC
  note: Inverter mode:
      |
      | m = 1.2
      | alpha = 0
      |
      | P = 1 kW x 3 phase
      | Q = 1 kVAr x3 phase
      | PF = 0.6
      | Vpu = 0.95
  note: Operation modes
  note: Rectif mode:
      |
      | m = 1
      | alpha = 228
      |
      | P = 975 kVA (DC)
  Means : Inport
  C1 : powerlib/Elements/Series RLC Branch  LConnTagsString=__new0  RConnTagsString=__new0  BranchType=C  Resistance=22.5  Inductance=1e-3  SetiL0=off  InitialCurrent=0  Capacitance=1200e-6  Setx0=off  InitialVoltage=150  Measurements=None
  Control of Inverter : Subsystem
      mask Display: image('Icons\FPGA.png');
  Ground1 : powerlib/Elements/Ground  LConnTagsString=a
  Scope : Scope
  Three-Phase Parallel RLC Branch1 : powerlib/Elements/Three-Phase Parallel RLC Branch  LConnTagsString=A|B|C  RConnTagsString=A|B|C  BranchType=C  Resistance=1  Inductance=1e-3  Capacitance=2.65e-6  Measurements=None
      settings: SourceProductBaseCode=PS
  Three-Phase Series RLC Branch1 : powerlib/Elements/Three-Phase Series RLC Branch  LConnTagsString=A|B|C  RConnTagsString=A|B|C  BranchType=RL  Resistance=2  Inductance=1e-2  Capacitance=15.5e-5  Measurements=None
  Universal Bridge1 : powerlib/Power Electronics/Universal Bridge  Arms=3  SnubberResistance=1e5  SnubberCapacitance=inf  Device=MOSFET / Diodes  Ron=1e-3  Lon=0  ForwardVoltages="[  0  0  ]"  ForwardVoltage=0  GTOparameters=[ 10e-6 , 20e-6 ]  IGBTparameters=[ 1e-6 , 2e-6 ]  Measurements=None  Measurements_2=None  converterType=Rectifier
  "a " : PMIOPort  Tag=PMCPort  Side=Left
  b : PMIOPort  Tag=PMCPort  Port=2  Side=Left
  c : PMIOPort  Tag=PMCPort  Port=3  Side=Left
  B1 + : PMIOPort  Port=4  Side=Right
  B1 - : PMIOPort  Port=5  Side=Right
  tag scope: Pulse=global
  wires:
  Control of Inverter/1(Pulses) -> Scope/1, [Pulse]
  [Pulse] -> Universal Bridge1/1
  Means/1 -> Control of Inverter/1(Means)
  connections:
  Three-Phase Series RLC Branch1/RConn1 -- Three-Phase Parallel RLC Branch1/LConn1 -- "a "/RConn1
  Three-Phase Parallel RLC Branch1/LConn2 -- Three-Phase Series RLC Branch1/RConn2 -- b/RConn1
  Three-Phase Parallel RLC Branch1/LConn3 -- Three-Phase Series RLC Branch1/RConn3 -- c/RConn1
  Ground1/LConn1 -- Three-Phase Parallel RLC Branch1/RConn3 -- Three-Phase Parallel RLC Branch1/RConn1 -- Three-Phase Parallel RLC Branch1/RConn2
  Universal Bridge1/LConn3 -- Three-Phase Series RLC Branch1/LConn3
  Three-Phase Series RLC Branch1/LConn2 -- Universal Bridge1/LConn2
  Universal Bridge1/LConn1 -- Three-Phase Series RLC Branch1/LConn1
  B1 +/RConn1 -- C1/LConn1 -- Universal Bridge1/RConn1
  B1 -/RConn1 -- C1/RConn1 -- Universal Bridge1/RConn2

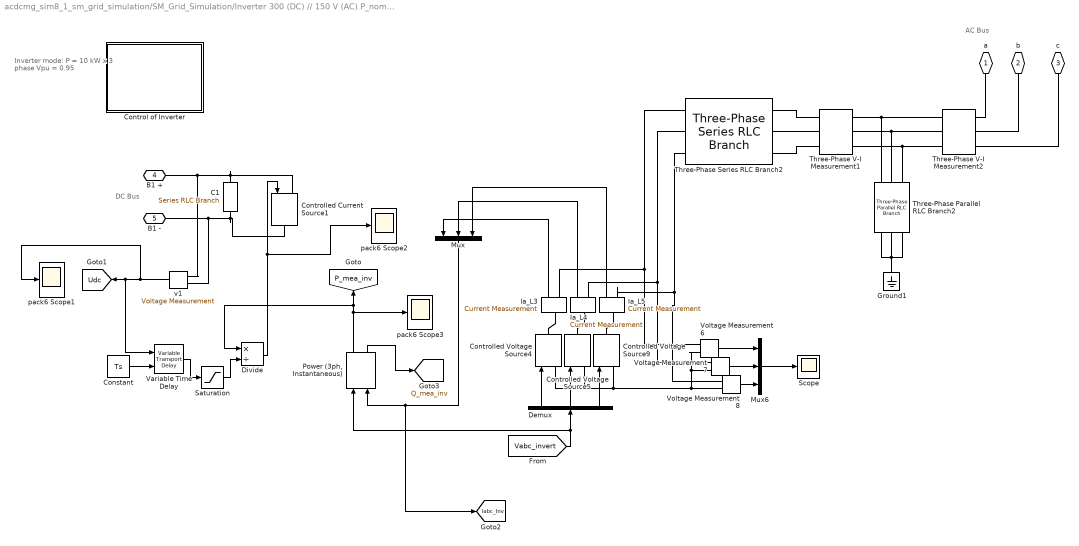
== system acdcmg_sim8_1_sm_grid_simulation/SM_Grid_Simulation/Inverter 300 (DC) // 150 V (AC) P_nom 10 kW4 ==
  note: DC Bus
  note: AC Bus
  note: Inverter mode:
      |
      | P = 10 kW x 3 phase
      | Vpu = 0.95
  C1 : powerlib/Elements/Series RLC Branch  LConnTagsString=__new0  RConnTagsString=__new0  BranchType=C  Resistance=22.5  Inductance=1e-3  SetiL0=off  InitialCurrent=0  Capacitance=1200e-6  Setx0=on  InitialVoltage=300  Measurements=None
  Constant : Constant  Value=Ts
  Control of Inverter : Subsystem
      mask Display: image('Icons\FPGA.png');
  Controlled Current Source1 : powerlib/Electrical Sources/Controlled Current Source  Initialize=on  Source_Type=AC  Amplitude=0  Phase=0  Frequency=0  Measurements=None
  Controlled Voltage Source4 : powerlib/Electrical Sources/Controlled Voltage Source  Initialize=off  Source_Type=AC  Amplitude=VnInv*sqrt(2)  Phase=0  Frequency=fn  Measurements=None
  Controlled Voltage Source5 : powerlib/Electrical Sources/Controlled Voltage Source  Initialize=off  Source_Type=AC  Amplitude=VnInv*sqrt(2)  Phase=0  Frequency=fn  Measurements=None
  Controlled Voltage Source9 : powerlib/Electrical Sources/Controlled Voltage Source  Initialize=off  Source_Type=AC  Amplitude=VnInv*sqrt(2)  Phase=0  Frequency=fn  Measurements=None
  Demux : Demux  Outputs=3
  Divide : Product  Inputs=*/
  Ground1 : powerlib/Elements/Ground  LConnTagsString=a
  Ia_L3 : powerlib/Measurements/Current Measurement  PhasorSimulation=off  OutputType=Complex  PSBequivalent=0
  Ia_L4 : powerlib/Measurements/Current Measurement  PhasorSimulation=off  OutputType=Complex  PSBequivalent=0
  Ia_L5 : powerlib/Measurements/Current Measurement  PhasorSimulation=off  OutputType=Complex  PSBequivalent=0
  Mux : Mux  Inputs=3
  Mux6 : Mux  Inputs=3
  "Power (3ph, Instantaneous)" : powerlib_meascontrol/Measurements/Power (3ph, Instantaneous)
  Saturation : Saturate  UpperLimit=inf  LowerLimit=0.01
  Scope : Scope
  Three-Phase Parallel RLC Branch2 : powerlib/Elements/Three-Phase Parallel RLC Branch  LConnTagsString=A|B|C  RConnTagsString=A|B|C  BranchType=C  Resistance=1  Inductance=1e-3  Capacitance=2.65e-6  Measurements=None
      settings: SourceProductBaseCode=PS
  Three-Phase Series RLC Branch2 : powerlib/Elements/Three-Phase Series RLC Branch  LConnTagsString=A|B|C  RConnTagsString=A|B|C  BranchType=RL  Resistance=0.02  Inductance=1e-2  Capacitance=15.5e-5  Measurements=None
  Three-Phase V-I Measurement1 : powerlib/Measurements/Three-Phase V-I Measurement  VoltageMeasurement=phase-to-ground  SetLabelV=on  LabelV=u  Vpu=off  VpuLL=off  CurrentMeasurement=yes  SetLabelI=on  LabelI=i  Ipu=off  Pbase=100e6  Vbase=500e3  OutputType=Complex  PhasorSimulation=off  PSBequivalent=0
  Three-Phase V-I Measurement2 : powerlib/Measurements/Three-Phase V-I Measurement  VoltageMeasurement=phase-to-ground  SetLabelV=on  LabelV=Vabc3  Vpu=off  VpuLL=off  CurrentMeasurement=yes  SetLabelI=on  LabelI=Iabc3  Ipu=off  Pbase=100e6  Vbase=500e3  OutputType=Complex  PhasorSimulation=off  PSBequivalent=0
  Variable Time Delay : VariableTransportDelay  MaximumDelay=2*Ts  InitialOutput=Ts
  Voltage Measurement6 : powerlib/Measurements/Voltage Measurement  PhasorSimulation=off  OutputType=Complex  PSBequivalent=0
  Voltage Measurement7 : powerlib/Measurements/Voltage Measurement  PhasorSimulation=off  OutputType=Complex  PSBequivalent=0
  Voltage Measurement8 : powerlib/Measurements/Voltage Measurement  PhasorSimulation=off  OutputType=Complex  PSBequivalent=0
  pack6 Scope1 : Scope
  pack6 Scope2 : Scope
  pack6 Scope3 : Scope
  v1 : powerlib/Measurements/Voltage Measurement  PhasorSimulation=off  OutputType=Complex  PSBequivalent=0
  "a " : PMIOPort  Tag=PMCPort  Side=Left
  b : PMIOPort  Tag=PMCPort  Port=2  Side=Left
  c : PMIOPort  Tag=PMCPort  Port=3  Side=Left
  B1 + : PMIOPort  Port=4  Side=Right
  B1 - : PMIOPort  Port=5  Side=Right
  tag scope: Iabc_Inv=global, P_mea_inv=global, Q_mea_inv=global, Udc=global
  wires:
  Voltage Measurement8/1 -> Mux6/3
  Mux6/1 -> Scope/1
  Voltage Measurement7/1 -> Mux6/2
  Voltage Measurement6/1 -> Mux6/1
  Demux/3 -> Controlled Voltage Source9/1
  Demux/2 -> Controlled Voltage Source5/1
  Demux/1 -> Controlled Voltage Source4/1
  Ia_L3/1 -> Mux/1
  Ia_L4/1 -> Mux/2
  Ia_L5/1 -> Mux/3
  Mux/1 -> [Iabc_Inv], "Power (3ph, Instantaneous)"/2
  "Power (3ph, Instantaneous)"/1 -> Divide/1, [P_mea_inv], pack6 Scope3/1
  Divide/1 -> pack6 Scope2/1, Controlled Current Source1/1
  [Vabc_invert] -> Demux/1, "Power (3ph, Instantaneous)"/1
  Constant/1 -> Variable Time Delay/2
  v1/1 -> pack6 Scope1/1, Variable Time Delay/1, [Udc]
  Variable Time Delay/1 -> Saturation/1
  Saturation/1 -> Divide/2
  "Power (3ph, Instantaneous)"/2 -> [Q_mea_inv]
  connections:
  Three-Phase V-I Measurement1/RConn1 -- Three-Phase V-I Measurement2/LConn1 -- Three-Phase Parallel RLC Branch2/LConn1
  Three-Phase Parallel RLC Branch2/LConn2 -- Three-Phase V-I Measurement2/LConn2 -- Three-Phase V-I Measurement1/RConn2
  Three-Phase V-I Measurement1/RConn3 -- Three-Phase V-I Measurement2/LConn3 -- Three-Phase Parallel RLC Branch2/LConn3
  Ground1/LConn1 -- Three-Phase Parallel RLC Branch2/RConn3 -- Three-Phase Parallel RLC Branch2/RConn1 -- Three-Phase Parallel RLC Branch2/RConn2
  Ia_L3/RConn1 -- Voltage Measurement6/LConn1 -- Three-Phase Series RLC Branch2/LConn1
  C1/LConn1 -- B1 +/RConn1 -- v1/LConn1 -- Controlled Current Source1/LConn1
  C1/RConn1 -- B1 -/RConn1 -- v1/LConn2 -- Controlled Current Source1/RConn1
  Three-Phase V-I Measurement1/LConn1 -- Three-Phase Series RLC Branch2/RConn1
  Three-Phase V-I Measurement1/LConn2 -- Three-Phase Series RLC Branch2/RConn2
  Three-Phase V-I Measurement1/LConn3 -- Three-Phase Series RLC Branch2/RConn3
  Three-Phase V-I Measurement2/RConn1 -- "a "/RConn1
  Three-Phase V-I Measurement2/RConn2 -- b/RConn1
  Three-Phase V-I Measurement2/RConn3 -- c/RConn1
  Controlled Voltage Source4/LConn1 -- Controlled Voltage Source5/LConn1 -- Controlled Voltage Source9/LConn1 -- Voltage Measurement6/LConn2 -- Voltage Measurement7/LConn2 -- Voltage Measurement8/LConn2
  Ia_L5/RConn1 -- Three-Phase Series RLC Branch2/LConn3 -- Voltage Measurement8/LConn1
  Three-Phase Series RLC Branch2/LConn2 -- Ia_L4/RConn1 -- Voltage Measurement7/LConn1
  Ia_L3/LConn1 -- Controlled Voltage Source4/RConn1
  Ia_L4/LConn1 -- Controlled Voltage Source5/RConn1
  Ia_L5/LConn1 -- Controlled Voltage Source9/RConn1

== system acdcmg_sim8_1_sm_grid_simulation/SM_Grid_Simulation/Main Grid 69 kV Inf ==
  note: Thevenin equivalent
  69kV 10000 MVA 1 : powerlib/Elements/Three-Phase Series RLC Branch  LConnTagsString=A|B|C  RConnTagsString=A|B|C  BranchType=RL  Resistance=69e3^2/10000e6/10  Inductance=69e3^2/10000e6/(2*pi*60)  Capacitance=1.0  Measurements=None
  Ground1 : powerlib/Elements/Ground  LConnTagsString=a
  Programmable Voltage Source1 : powerlib/Electrical Sources/Three-Phase Programmable Voltage Source  PositiveSequence="[69e3 0  60]"  VariationEntity=None  VariationType=Table of time-amplitude pairs  VariationTypeAlt=Step  VariationStep=-0.3  VariationRate=0.5  VariationMagnitude=0.4  VariationFrequency=2  VariationTiming=[0.1 1.2]  VariationPhaseA=off  Amplitudes=[1]  TimeValues=[0]  HarmonicGeneration=off  HarmonicA=[3 0.2 -25 0]  HarmonicB="[2 0.15  35 2]"  Timing="[0.1  0.6]"  BusType=swing  Pref=500  Qref=0  Qmin=-inf  Qmax=inf
  C : PMIOPort  Side=Right
  B : PMIOPort  Port=2  Side=Right
  A : PMIOPort  Port=3  Side=Right
  connections:
  Programmable Voltage Source1/RConn3 -- 69kV 10000 MVA 1/LConn3
  Ground1/LConn1 -- Programmable Voltage Source1/LConn1
  Programmable Voltage Source1/RConn2 -- 69kV 10000 MVA 1/LConn2
  69kV 10000 MVA 1/LConn1 -- Programmable Voltage Source1/RConn1
  69kV 10000 MVA 1/RConn3 -- C/RConn1
  69kV 10000 MVA 1/RConn2 -- B/RConn1
  69kV 10000 MVA 1/RConn1 -- A/RConn1

== system acdcmg_sim8_1_sm_grid_simulation/SM_Grid_Simulation/Non Linear AC  Load 9 ==
  Display : Display
  Mean : powerlib_meascontrol/Measurements/Mean  Freq=100  Vinit=0  Ts=0
  No lineal AC Load 320Kw : powerlib/Power Electronics/Universal Bridge  Arms=3  SnubberResistance=1e5  SnubberCapacitance=inf  Device=Thyristors  Ron=1e-3  Lon=0  ForwardVoltages="[  0  0  ]"  ForwardVoltage=0  GTOparameters=[ 10e-6 , 20e-6 ]  IGBTparameters=[ 1e-6 , 2e-6 ]  Measurements=None  Measurements_2=None  converterType=Rectifier
  PWM Generator (2-Level) : powerlib_meascontrol/Pulse & Signal Generators/PWM Generator (2-Level)  ModulatorType=Three-phase bridge (6 pulses)  ModulatorMode=Unsynchronized  Fc=4080  Pc=0  nF=27  MinMax="[ -1  1 ]"  SamplingTechnique=Natural  ModulatingSignals=on  m=0.8  Freq=Fnom  Phase=-30  Ts=0  ShowCarrierOutport=off
  RL : powerlib/Elements/Series RLC Branch  LConnTagsString=__new0  RConnTagsString=__new0  BranchType=R  Resistance=R_Load_9  Inductance=5e-3  SetiL0=off  InitialCurrent=0  Capacitance=1e-6  Setx0=off  InitialVoltage=0  Measurements=None
  RL1 : powerlib/Elements/Series RLC Branch  LConnTagsString=__new0  RConnTagsString=__new0  BranchType=C  Resistance=1  Inductance=5e-3  SetiL0=off  InitialCurrent=0  Capacitance=10e-6  Setx0=off  InitialVoltage=0  Measurements=None
  "Vdc " : powerlib/Measurements/Voltage Measurement  Tag=PoWeRsYsTeMmEaSuReMeNt  PhasorSimulation=off  OutputType=Magnitude  PSBequivalent=0
  A : PMIOPort  Tag=PMCPort  Side=Left
  B : PMIOPort  Tag=PMCPort  Port=2  Side=Left
  C : PMIOPort  Tag=PMCPort  Port=3  Side=Left
  wires:
  PWM Generator (2-Level)/1 -> No lineal AC Load 320Kw/1
  "Vdc "/1 -> Mean/1
  Mean/1 -> Display/1
  connections:
  No lineal AC Load 320Kw/RConn1 -- "Vdc "/LConn1 -- RL1/LConn1 -- RL/LConn1
  A/RConn1 -- No lineal AC Load 320Kw/LConn1
  C/RConn1 -- No lineal AC Load 320Kw/LConn3
  B/RConn1 -- No lineal AC Load 320Kw/LConn2
  No lineal AC Load 320Kw/RConn2 -- "Vdc "/LConn2 -- RL1/RConn1 -- RL/RConn1

== system acdcmg_sim8_1_sm_grid_simulation/SM_Grid_Simulation/OpComm1 ==
  Demux : Demux  Outputs="[1  1  1  1  1  1  1  1]"
  Receive : opal_lib/Communication/OpRecPar FromNT  Data_width=8  InitialConditions=[0;1;1;0;1;1;1;1]
  busStruct : Subsystem
  Out1 : Outport
  Out2 : Outport  Port=2
  Out3 : Outport  Port=3
  Out4 : Outport  Port=4
  Out5 : Outport  Port=5
  Out6 : Outport  Port=6
  Out7 : Outport  Port=7
  Out8 : Outport  Port=8
  wires:
  Demux/8 -> busStruct/8(In8)
  Demux/7 -> busStruct/7(In7)
  Demux/6 -> busStruct/6(In6)
  Demux/5 -> busStruct/5(In5)
  Demux/4 -> busStruct/4(In4)
  Demux/3 -> busStruct/3(In3)
  Demux/2 -> busStruct/2(In2)
  Demux/1 -> busStruct/1(In1)
  busStruct/8(Out8) -> Out8/1
  busStruct/7(Out7) -> Out7/1
  busStruct/6(Out6) -> Out6/1
  busStruct/5(Out5) -> Out5/1
  busStruct/4(Out4) -> Out4/1
  busStruct/3(Out3) -> Out3/1
  busStruct/2(Out2) -> Out2/1
  busStruct/1(Out1) -> Out1/1
  Receive/1 -> Demux/1

== system acdcmg_sim8_1_sm_grid_simulation/SM_Grid_Simulation/PV Subsystem ==
  Bus Selector : BusSelector  OutputSignals=V_PV,I_PV  OutputAsBus=on
  Diode1 : powerlib/Power Electronics/Diode  Ron=0.001  Lon=0  Vf=0.7  IC=0  UseSnubber=off  Rs=1e5  Cs=1e5  Measurements=on
  Display : Display
  Ground : powerlib/Elements/Ground  LConnTagsString=a
      settings: SourceProductName=Simscape Electrical
  I : powerlib/Measurements/Current Measurement  PhasorSimulation=off  OutputType=Complex  PSBequivalent=0
  Ir1 : Constant  Value=1000
  PV Array : re_lib/Solar/PV Array  Npar=40  Nser=10  PlotType=array @ 1000 W/m2 & specified temperatures  S_vec="[ 1000  500  100 ]"  Temp_C_vec="[ 45 25  ]"  ModuleName=1Soltech 1STH-215-P  PlotWhenSelected=off  Pm=213.15  Ncell=60  Voc=36.3  Isc=7.84  Vm=29  Im=7.35  beta_Voc_pc=-0.36099  alpha_Isc_pc=0.102  beta_Voc=-0.13104  alpha_Isc=0.007997  IL=7.8649  I0=2.9259e-10  nI=0.98117  Rsh=313.3991  Rs=0.39383  BAL=on  Tc=1e-6  Tfilter=5e-5
      settings: SourceProductName=Simscape Electrical
  Rate Limiter : RateLimiter  SampleTimeMode=inherited  InitialCondition=1
  Saturation : Saturate  UpperLimit=26
  Scope : Scope  NumInputPorts=2
  Scope1 : Scope
  Temp C : Constant  Value=25
  V : powerlib/Measurements/Voltage Measurement  PhasorSimulation=off  OutputType=Complex  PSBequivalent=0
  T2+ : PMIOPort  Side=Right
  T2- : PMIOPort  Port=2  Side=Right
  tag scope: m_PV=global
  wires:
  V/1 -> Display/1, Scope/2, [V]
  Diode1/1 -> [VI_D]
  Temp C/1 -> Saturation/1
  PV Array/1 -> Scope1/1, [m_PV], Bus Selector/1
  Ir1/1 -> Rate Limiter/1
  Bus Selector/1 -> [VI_PV]
  I/1 -> Scope/1, [I]
  Saturation/1 -> PV Array/2
  Rate Limiter/1 -> PV Array/1
  connections:
  V/LConn1 -- I/LConn1 -- PV Array/RConn1 -- Diode1/RConn1
  T2-/RConn1 -- Ground/LConn1 -- V/LConn2 -- PV Array/RConn2 -- Diode1/LConn1
  I/RConn1 -- T2+/RConn1

== system acdcmg_sim8_1_sm_grid_simulation/SM_Grid_Simulation/Subsystem ==
